simulink model "skyhooksemiMR"  (R2016a)
settings: Solver=VariableStepAuto  StartTime=0.0  StopTime=10.0  RelTol=1e-3
undefined symbols (not defined in the file): b1, k1, k2, m1, m2
settings Model: Creator=mm395  LastModifiedBy=mm395

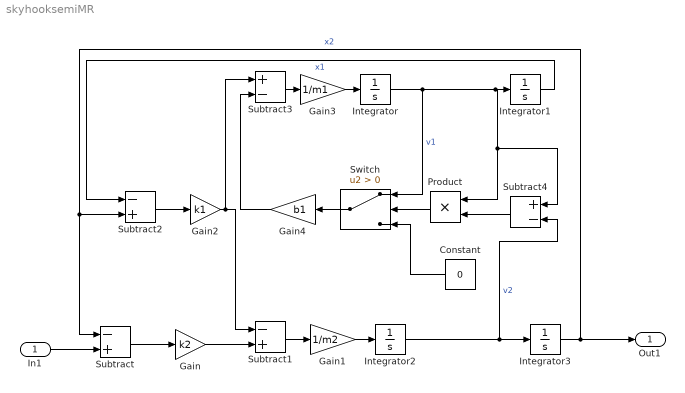
== system skyhooksemiMR ==
  In1 : Inport
  Constant : Constant  Value=0
  Gain : Gain  Gain=k2
  Gain1 : Gain  Gain=1/m2
  Gain2 : Gain  Gain=k1
  Gain3 : Gain  Gain=1/m1
  Gain4 : Gain  Gain=b1
  Integrator{,1..3} (4 alike) : Integrator
  Product : Product
  Subtract : Sum  Inputs=-+
  Subtract1 : Sum  Inputs=-+
  Subtract2 : Sum  Inputs=-+
  Subtract3 : Sum  Inputs=+-
  Subtract4 : Sum  Inputs=+-
  Switch : Switch  Criteria=u2 > Threshold
  Out1 : Outport
  wires:
  In1/1 -> Subtract/2
  Subtract/1 -> Gain/1
  Gain/1 -> Subtract1/2
  Subtract1/1 -> Gain1/1
  Integrator3/1 -> Out1/1, Subtract/1, Subtract2/2  "x2"
  Subtract2/1 -> Gain2/1
  Gain2/1 -> Subtract3/1, Subtract1/1
  Subtract3/1 -> Gain3/1
  Gain3/1 -> Integrator/1
  Integrator/1 -> Switch/1, Product/1, Subtract4/1, Integrator1/1  "v1"
  Integrator2/1 -> Subtract4/2, Integrator3/1  "v2"
  Gain1/1 -> Integrator2/1
  Integrator1/1 -> Subtract2/1  "x1"
  Subtract4/1 -> Product/2
  Product/1 -> Switch/2
  Switch/1 -> Gain4/1
  Gain4/1 -> Subtract3/2
  Constant/1 -> Switch/3
